simulink library "Word_Multiplexers_Lib"  (Simulink 8.7)
settings: Solver=ode45  StartTime=0.0  StopTime=10.0  RelTol=1e-3
(part 3 of 3)

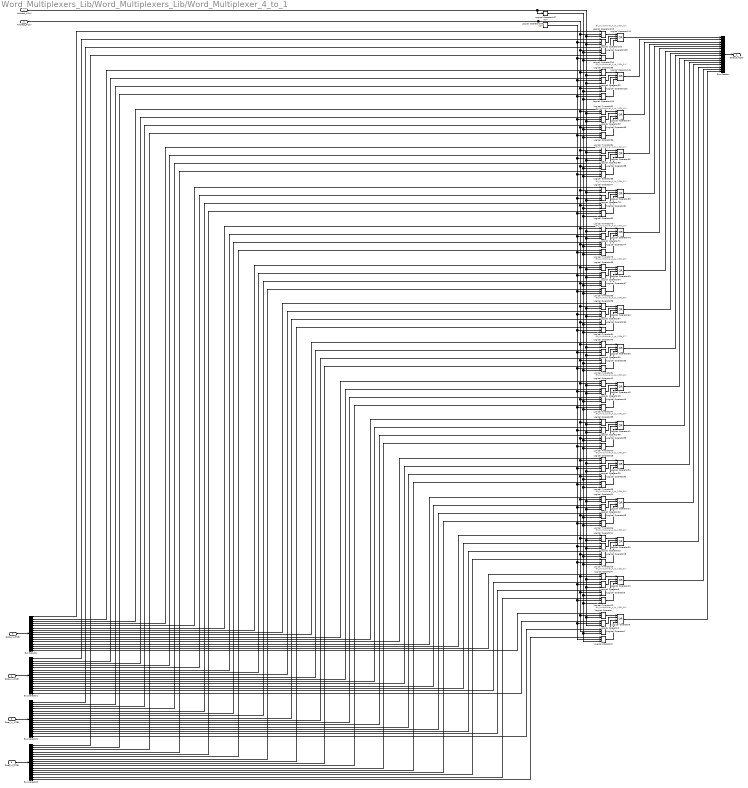
== system Word_Multiplexers_Lib/Word_Multiplexers_Lib/Word_Multiplexer_4_to_1 ==
  note: Bit_Multiplexer_4_to_1(Bit_15)
  note: Bit_Multiplexer_4_to_1(Bit_14)
  note: Bit_Multiplexer_4_to_1(Bit_13)
  note: Bit_Multiplexer_4_to_1(Bit_12)
  note: Bit_Multiplexer_4_to_1(Bit_11)
  note: Bit_Multiplexer_4_to_1(Bit_10)
  note: Bit_Multiplexer_4_to_1(Bit_09)
  note: Bit_Multiplexer_4_to_1(Bit_08)
  note: Bit_Multiplexer_4_to_1(Bit_07)
  note: Bit_Multiplexer_4_to_1(Bit_06)
  note: Bit_Multiplexer_4_to_1(Bit_05)
  note: Bit_Multiplexer_4_to_1(Bit_04)
  note: Bit_Multiplexer_4_to_1(Bit_03)
  note: Bit_Multiplexer_4_to_1(Bit_02)
  note: Bit_Multiplexer_4_to_1(Bit_01)
  note: Bit_Multiplexer_4_to_1(Bit_00)
  Address_1(1b) : Inport
  Address_0(1b) : Inport  Port=2
  Data_In_3(2B) : Inport  Port=3
  Data_In_2(2B) : Inport  Port=4
  Data_In_1(2B) : Inport  Port=5
  Data_In_0(2B) : Inport  Port=6
  Bus Creator : BusCreator  Inputs=16
  Bus Selector{,1..3} (4 alike) : BusSelector  OutputSignals=signal1,signal2,signal3,signal4,signal5,signal6,signal7,signal8,signal9,signal10,signal11,signal12,signal13,signal14,signal15,signal16
  Logical Operator{,1..5,9..10,14..15,18..19,21..22,25..26,28..29,32..33,35..36,39..40,42..43,46..47,49..50,53..54,56..57,60..61,63..64,67..68,70..71,74..75,77..78,81..82,84..85,88..89,91..92,95..96,98..99,102..103,105..106,109..110} (64 alike) : Logic  Inputs=3  IconShape=distinctive  AllPortsSameDT=off  OutDataTypeStr=boolean
  Logical Operator{8,13,20,27,34,41,48,55,62,69,76,83,90,97,104,111} (16 alike) : Logic  Operator=OR  Inputs=4  IconShape=distinctive  OutDataTypeStr=boolean
  Logical Operator107 : Logic  Operator=NOT  Inputs=4  IconShape=distinctive  AllPortsSameDT=off  OutDataTypeStr=boolean
  Logical Operator108 : Logic  Operator=NOT  Inputs=4  IconShape=distinctive  AllPortsSameDT=off  OutDataTypeStr=boolean
  Data_Out(2B) : Outport
  wires:
  Bus Creator/1 -> Data_Out(2B)/1
  Logical Operator34/1 -> Bus Creator/12
  Logical Operator41/1 -> Bus Creator/11
  Logical Operator48/1 -> Bus Creator/10
  Logical Operator55/1 -> Bus Creator/9
  Logical Operator27/1 -> Bus Creator/13
  Logical Operator20/1 -> Bus Creator/14
  Logical Operator13/1 -> Bus Creator/15
  Logical Operator8/1 -> Bus Creator/16
  Data_In_3(2B)/1 -> Bus Selector/1
  Data_In_2(2B)/1 -> Bus Selector1/1
  Data_In_1(2B)/1 -> Bus Selector2/1
  Data_In_0(2B)/1 -> Bus Selector3/1
  Logical Operator62/1 -> Bus Creator/8
  Logical Operator69/1 -> Bus Creator/7
  Logical Operator76/1 -> Bus Creator/6
  Logical Operator83/1 -> Bus Creator/5
  Logical Operator90/1 -> Bus Creator/4
  Logical Operator97/1 -> Bus Creator/3
  Logical Operator104/1 -> Bus Creator/2
  Logical Operator111/1 -> Bus Creator/1
  Logical Operator108/1 -> Logical Operator106/2, Logical Operator57/2, Logical Operator43/2, Logical Operator1/2, Logical Operator3/2, Logical Operator10/2, Logical Operator5/2, Logical Operator19/2, Logical Operator15/2, Logical Operator26/2, Logical Operator22/2, Logical Operator33/2, Logical Operator29/2, Logical Operator40/2, Logical Operator36/2, Logical Operator47/2, Logical Operator54/2, Logical Operator50/2, Logical Operator61/2, Logical Operator68/2, Logical Operator64/2, Logical Operator75/2, Logical Operator71/2, Logical Operator82/2, Logical Operator78/2, Logical Operator89/2, Logical Operator85/2, Logical Operator96/2, Logical Operator92/2, Logical Operator103/2, Logical Operator99/2, Logical Operator110/2
  Logical Operator107/1 -> Logical Operator109/3, Logical Operator60/3, Logical Operator46/3, Logical Operator10/3, Logical Operator2/3, Logical Operator3/3, Logical Operator9/3, Logical Operator19/3, Logical Operator18/3, Logical Operator26/3, Logical Operator25/3, Logical Operator33/3, Logical Operator32/3, Logical Operator40/3, Logical Operator39/3, Logical Operator47/3, Logical Operator54/3, Logical Operator53/3, Logical Operator61/3, Logical Operator68/3, Logical Operator67/3, Logical Operator75/3, Logical Operator74/3, Logical Operator82/3, Logical Operator81/3, Logical Operator89/3, Logical Operator88/3, Logical Operator96/3, Logical Operator95/3, Logical Operator103/3, Logical Operator102/3, Logical Operator110/3
  Bus Selector/16 -> Logical Operator/1  "<signal16>"
  Bus Selector1/16 -> Logical Operator1/1  "<signal16>"
  Bus Selector2/16 -> Logical Operator2/1  "<signal16>"
  Bus Selector3/16 -> Logical Operator3/1  "<signal16>"
  Logical Operator3/1 -> Logical Operator8/4
  Logical Operator2/1 -> Logical Operator8/3
  Logical Operator1/1 -> Logical Operator8/2
  Logical Operator/1 -> Logical Operator8/1
  Bus Selector/15 -> Logical Operator4/1  "<signal15>"
  Bus Selector1/15 -> Logical Operator5/1  "<signal15>"
  Bus Selector2/15 -> Logical Operator9/1  "<signal15>"
  Bus Selector3/15 -> Logical Operator10/1  "<signal15>"
  Logical Operator10/1 -> Logical Operator13/4
  Logical Operator9/1 -> Logical Operator13/3
  Logical Operator5/1 -> Logical Operator13/2
  Logical Operator4/1 -> Logical Operator13/1
  Bus Selector/14 -> Logical Operator14/1  "<signal14>"
  Bus Selector1/14 -> Logical Operator15/1  "<signal14>"
  Bus Selector2/14 -> Logical Operator18/1  "<signal14>"
  Bus Selector3/14 -> Logical Operator19/1  "<signal14>"
  Logical Operator19/1 -> Logical Operator20/4
  Logical Operator18/1 -> Logical Operator20/3
  Logical Operator15/1 -> Logical Operator20/2
  Logical Operator14/1 -> Logical Operator20/1
  Bus Selector/13 -> Logical Operator21/1  "<signal13>"
  Bus Selector1/13 -> Logical Operator22/1  "<signal13>"
  Bus Selector2/13 -> Logical Operator25/1  "<signal13>"
  Bus Selector3/13 -> Logical Operator26/1  "<signal13>"
  Logical Operator26/1 -> Logical Operator27/4
  Logical Operator25/1 -> Logical Operator27/3
  Logical Operator22/1 -> Logical Operator27/2
  Logical Operator21/1 -> Logical Operator27/1
  Bus Selector/12 -> Logical Operator28/1  "<signal12>"
  Bus Selector1/12 -> Logical Operator29/1  "<signal12>"
  Bus Selector2/12 -> Logical Operator32/1  "<signal12>"
  Bus Selector3/12 -> Logical Operator33/1  "<signal12>"
  Logical Operator33/1 -> Logical Operator34/4
  Logical Operator32/1 -> Logical Operator34/3
  Logical Operator29/1 -> Logical Operator34/2
  Logical Operator28/1 -> Logical Operator34/1
  Bus Selector/11 -> Logical Operator35/1  "<signal11>"
  Bus Selector1/11 -> Logical Operator36/1  "<signal11>"
  Bus Selector2/11 -> Logical Operator39/1  "<signal11>"
  Bus Selector3/11 -> Logical Operator40/1  "<signal11>"
  Logical Operator40/1 -> Logical Operator41/4
  Logical Operator39/1 -> Logical Operator41/3
  Logical Operator36/1 -> Logical Operator41/2
  Logical Operator35/1 -> Logical Operator41/1
  Bus Selector/10 -> Logical Operator42/1  "<signal10>"
  Bus Selector1/10 -> Logical Operator43/1  "<signal10>"
  Bus Selector2/10 -> Logical Operator46/1  "<signal10>"
  Bus Selector3/10 -> Logical Operator47/1  "<signal10>"
  Logical Operator47/1 -> Logical Operator48/4
  Logical Operator46/1 -> Logical Operator48/3
  Logical Operator43/1 -> Logical Operator48/2
  Logical Operator42/1 -> Logical Operator48/1
  Bus Selector/9 -> Logical Operator49/1  "<signal9>"
  Bus Selector1/9 -> Logical Operator50/1  "<signal9>"
  Bus Selector2/9 -> Logical Operator53/1  "<signal9>"
  Bus Selector3/9 -> Logical Operator54/1  "<signal9>"
  Logical Operator54/1 -> Logical Operator55/4
  Logical Operator53/1 -> Logical Operator55/3
  Logical Operator50/1 -> Logical Operator55/2
  Logical Operator49/1 -> Logical Operator55/1
  Bus Selector/8 -> Logical Operator56/1  "<signal8>"
  Bus Selector1/8 -> Logical Operator57/1  "<signal8>"
  Bus Selector2/8 -> Logical Operator60/1  "<signal8>"
  Bus Selector3/8 -> Logical Operator61/1  "<signal8>"
  Logical Operator61/1 -> Logical Operator62/4
  Logical Operator60/1 -> Logical Operator62/3
  Logical Operator57/1 -> Logical Operator62/2
  Logical Operator56/1 -> Logical Operator62/1
  Bus Selector/7 -> Logical Operator63/1  "<signal7>"
  Bus Selector1/7 -> Logical Operator64/1  "<signal7>"
  Bus Selector2/7 -> Logical Operator67/1  "<signal7>"
  Bus Selector3/7 -> Logical Operator68/1  "<signal7>"
  Logical Operator68/1 -> Logical Operator69/4
  Logical Operator67/1 -> Logical Operator69/3
  Logical Operator64/1 -> Logical Operator69/2
  Logical Operator63/1 -> Logical Operator69/1
  Bus Selector/6 -> Logical Operator70/1  "<signal6>"
  Bus Selector1/6 -> Logical Operator71/1  "<signal6>"
  Bus Selector2/6 -> Logical Operator74/1  "<signal6>"
  Bus Selector3/6 -> Logical Operator75/1  "<signal6>"
  Logical Operator75/1 -> Logical Operator76/4
  Logical Operator74/1 -> Logical Operator76/3
  Logical Operator71/1 -> Logical Operator76/2
  Logical Operator70/1 -> Logical Operator76/1
  Bus Selector/5 -> Logical Operator77/1  "<signal5>"
  Bus Selector1/5 -> Logical Operator78/1  "<signal5>"
  Bus Selector2/5 -> Logical Operator81/1  "<signal5>"
  Bus Selector3/5 -> Logical Operator82/1  "<signal5>"
  Logical Operator82/1 -> Logical Operator83/4
  Logical Operator81/1 -> Logical Operator83/3
  Logical Operator78/1 -> Logical Operator83/2
  Logical Operator77/1 -> Logical Operator83/1
  Bus Selector/4 -> Logical Operator84/1  "<signal4>"
  Bus Selector1/4 -> Logical Operator85/1  "<signal4>"
  Bus Selector2/4 -> Logical Operator88/1  "<signal4>"
  Bus Selector3/4 -> Logical Operator89/1  "<signal4>"
  Logical Operator89/1 -> Logical Operator90/4
  Logical Operator88/1 -> Logical Operator90/3
  Logical Operator85/1 -> Logical Operator90/2
  Logical Operator84/1 -> Logical Operator90/1
  Bus Selector/3 -> Logical Operator91/1  "<signal3>"
  Bus Selector1/3 -> Logical Operator92/1  "<signal3>"
  Bus Selector2/3 -> Logical Operator95/1  "<signal3>"
  Bus Selector3/3 -> Logical Operator96/1  "<signal3>"
  Logical Operator96/1 -> Logical Operator97/4
  Logical Operator95/1 -> Logical Operator97/3
  Logical Operator92/1 -> Logical Operator97/2
  Logical Operator91/1 -> Logical Operator97/1
  Bus Selector/2 -> Logical Operator98/1  "<signal2>"
  Bus Selector1/2 -> Logical Operator99/1  "<signal2>"
  Bus Selector2/2 -> Logical Operator102/1  "<signal2>"
  Bus Selector3/2 -> Logical Operator103/1  "<signal2>"
  Logical Operator103/1 -> Logical Operator104/4
  Logical Operator102/1 -> Logical Operator104/3
  Logical Operator99/1 -> Logical Operator104/2
  Logical Operator98/1 -> Logical Operator104/1
  Address_0(1b)/1 -> Logical Operator105/2, Logical Operator56/2, Logical Operator42/2, Logical Operator/2, Logical Operator2/2, Logical Operator9/2, Logical Operator4/2, Logical Operator18/2, Logical Operator14/2, Logical Operator25/2, Logical Operator21/2, Logical Operator32/2, Logical Operator28/2, Logical Operator39/2, Logical Operator35/2, Logical Operator46/2, Logical Operator53/2, Logical Operator49/2, Logical Operator60/2, Logical Operator67/2, Logical Operator63/2, Logical Operator74/2, Logical Operator70/2, Logical Operator81/2, Logical Operator77/2, Logical Operator88/2, Logical Operator84/2, Logical Operator95/2, Logical Operator91/2, Logical Operator102/2, Logical Operator98/2, Logical Operator109/2, Logical Operator108/1
  Address_1(1b)/1 -> Logical Operator107/1, Logical Operator105/3, Logical Operator56/3, Logical Operator42/3, Logical Operator/3, Logical Operator1/3, Logical Operator5/3, Logical Operator4/3, Logical Operator15/3, Logical Operator14/3, Logical Operator22/3, Logical Operator21/3, Logical Operator29/3, Logical Operator28/3, Logical Operator36/3, Logical Operator35/3, Logical Operator43/3, Logical Operator50/3, Logical Operator49/3, Logical Operator57/3, Logical Operator64/3, Logical Operator63/3, Logical Operator71/3, Logical Operator70/3, Logical Operator78/3, Logical Operator77/3, Logical Operator85/3, Logical Operator84/3, Logical Operator92/3, Logical Operator91/3, Logical Operator99/3, Logical Operator98/3, Logical Operator106/3
  Bus Selector/1 -> Logical Operator105/1  "<signal1>"
  Bus Selector1/1 -> Logical Operator106/1  "<signal1>"
  Bus Selector2/1 -> Logical Operator109/1  "<signal1>"
  Bus Selector3/1 -> Logical Operator110/1  "<signal1>"
  Logical Operator110/1 -> Logical Operator111/4
  Logical Operator109/1 -> Logical Operator111/3
  Logical Operator106/1 -> Logical Operator111/2
  Logical Operator105/1 -> Logical Operator111/1

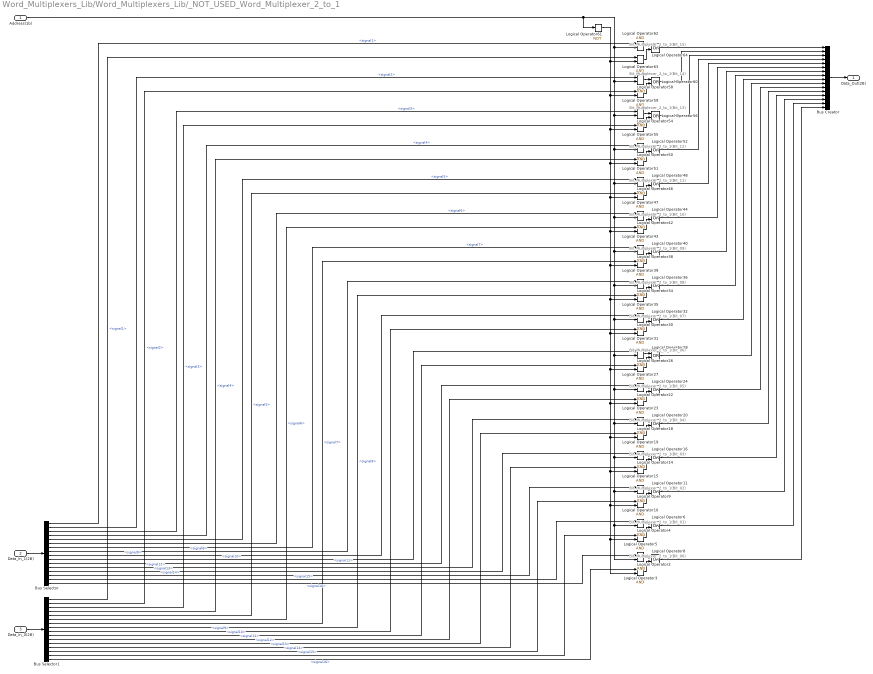
== system Word_Multiplexers_Lib/Word_Multiplexers_Lib/_NOT_USED_Word_Multiplexer_2_to_1 ==
  note: Bit_Multiplexer_2_to_1(Bit_15)
  note: Bit_Multiplexer_2_to_1(Bit_14)
  note: Bit_Multiplexer_2_to_1(Bit_13)
  note: Bit_Multiplexer_2_to_1(Bit_12)
  note: Bit_Multiplexer_2_to_1(Bit_11)
  note: Bit_Multiplexer_2_to_1(Bit_10)
  note: Bit_Multiplexer_2_to_1(Bit_09)
  note: Bit_Multiplexer_2_to_1(Bit_08)
  note: Bit_Multiplexer_2_to_1(Bit_07)
  note: Bit_Multiplexer_2_to_1(Bit_06)
  note: Bit_Multiplexer_2_to_1(Bit_05)
  note: Bit_Multiplexer_2_to_1(Bit_04)
  note: Bit_Multiplexer_2_to_1(Bit_03)
  note: Bit_Multiplexer_2_to_1(Bit_02)
  note: Bit_Multiplexer_2_to_1(Bit_01)
  note: Bit_Multiplexer_2_to_1(Bit_00)
  Address(1b) : Inport
  Data_In_1(2B) : Inport  Port=2
  Data_In_0(2B) : Inport  Port=3
  Bus Creator : BusCreator  Inputs=16
  Bus Selector : BusSelector  OutputSignals=signal1,signal2,signal3,signal4,signal5,signal6,signal7,signal8,signal9,signal10,signal11,signal12,signal13,signal14,signal15,signal16
  Bus Selector1 : BusSelector  OutputSignals=signal1,signal2,signal3,signal4,signal5,signal6,signal7,signal8,signal9,signal10,signal11,signal12,signal13,signal14,signal15,signal16
  Logical Operator{2..5,9..10,14..15,18..19,22..23,26..27,30..31,34..35,38..39,42..43,46..47,50..51,54..55,58..59,62..63} (32 alike) : Logic  IconShape=distinctive  AllPortsSameDT=off  OutDataTypeStr=boolean
  Logical Operator{6,8,11,16,20,24,28,32,36,40,44,48,52,56,60,64} (16 alike) : Logic  Operator=OR  IconShape=distinctive  OutDataTypeStr=boolean
  Logical Operator61 : Logic  Operator=NOT  Inputs=4  IconShape=distinctive  AllPortsSameDT=off  OutDataTypeStr=boolean
  Data_Out(2B) : Outport
  wires:
  Logical Operator64/1 -> Bus Creator/1
  Logical Operator60/1 -> Bus Creator/2
  Logical Operator56/1 -> Bus Creator/3
  Logical Operator52/1 -> Bus Creator/4
  Logical Operator48/1 -> Bus Creator/5
  Logical Operator44/1 -> Bus Creator/6
  Logical Operator40/1 -> Bus Creator/7
  Logical Operator36/1 -> Bus Creator/8
  Data_In_0(2B)/1 -> Bus Selector1/1
  Data_In_1(2B)/1 -> Bus Selector/1
  Logical Operator8/1 -> Bus Creator/16
  Logical Operator6/1 -> Bus Creator/15
  Logical Operator11/1 -> Bus Creator/14
  Logical Operator16/1 -> Bus Creator/13
  Logical Operator32/1 -> Bus Creator/9
  Logical Operator28/1 -> Bus Creator/10
  Logical Operator24/1 -> Bus Creator/11
  Logical Operator20/1 -> Bus Creator/12
  Bus Creator/1 -> Data_Out(2B)/1
  Logical Operator61/1 -> Logical Operator3/2, Logical Operator5/2, Logical Operator10/2, Logical Operator15/2, Logical Operator19/2, Logical Operator23/2, Logical Operator27/2, Logical Operator31/2, Logical Operator35/2, Logical Operator39/2, Logical Operator43/2, Logical Operator47/2, Logical Operator51/2, Logical Operator55/2, Logical Operator59/2, Logical Operator63/2
  Bus Selector/16 -> Logical Operator2/1  "<signal16>"
  Bus Selector1/16 -> Logical Operator3/1  "<signal16>"
  Logical Operator3/1 -> Logical Operator8/2
  Logical Operator2/1 -> Logical Operator8/1
  Bus Selector/15 -> Logical Operator4/1  "<signal15>"
  Bus Selector1/15 -> Logical Operator5/1  "<signal15>"
  Logical Operator5/1 -> Logical Operator6/2
  Logical Operator4/1 -> Logical Operator6/1
  Bus Selector/14 -> Logical Operator9/1  "<signal14>"
  Bus Selector1/14 -> Logical Operator10/1  "<signal14>"
  Logical Operator10/1 -> Logical Operator11/2
  Logical Operator9/1 -> Logical Operator11/1
  Bus Selector/13 -> Logical Operator14/1  "<signal13>"
  Bus Selector1/13 -> Logical Operator15/1  "<signal13>"
  Logical Operator15/1 -> Logical Operator16/2
  Logical Operator14/1 -> Logical Operator16/1
  Bus Selector/12 -> Logical Operator18/1  "<signal12>"
  Bus Selector1/12 -> Logical Operator19/1  "<signal12>"
  Logical Operator19/1 -> Logical Operator20/2
  Logical Operator18/1 -> Logical Operator20/1
  Bus Selector/11 -> Logical Operator22/1  "<signal11>"
  Bus Selector1/11 -> Logical Operator23/1  "<signal11>"
  Logical Operator23/1 -> Logical Operator24/2
  Logical Operator22/1 -> Logical Operator24/1
  Bus Selector/10 -> Logical Operator26/1  "<signal10>"
  Bus Selector1/10 -> Logical Operator27/1  "<signal10>"
  Logical Operator27/1 -> Logical Operator28/2
  Logical Operator26/1 -> Logical Operator28/1
  Bus Selector/9 -> Logical Operator30/1  "<signal9>"
  Bus Selector1/9 -> Logical Operator31/1  "<signal9>"
  Logical Operator31/1 -> Logical Operator32/2
  Logical Operator30/1 -> Logical Operator32/1
  Bus Selector/8 -> Logical Operator34/1  "<signal8>"
  Bus Selector1/8 -> Logical Operator35/1  "<signal8>"
  Logical Operator35/1 -> Logical Operator36/2
  Logical Operator34/1 -> Logical Operator36/1
  Bus Selector/7 -> Logical Operator38/1  "<signal7>"
  Bus Selector1/7 -> Logical Operator39/1  "<signal7>"
  Logical Operator39/1 -> Logical Operator40/2
  Logical Operator38/1 -> Logical Operator40/1
  Bus Selector/6 -> Logical Operator42/1  "<signal6>"
  Bus Selector1/6 -> Logical Operator43/1  "<signal6>"
  Logical Operator43/1 -> Logical Operator44/2
  Logical Operator42/1 -> Logical Operator44/1
  Bus Selector/5 -> Logical Operator46/1  "<signal5>"
  Bus Selector1/5 -> Logical Operator47/1  "<signal5>"
  Logical Operator47/1 -> Logical Operator48/2
  Logical Operator46/1 -> Logical Operator48/1
  Bus Selector/4 -> Logical Operator50/1  "<signal4>"
  Bus Selector1/4 -> Logical Operator51/1  "<signal4>"
  Logical Operator51/1 -> Logical Operator52/2
  Logical Operator50/1 -> Logical Operator52/1
  Bus Selector/3 -> Logical Operator54/1  "<signal3>"
  Bus Selector1/3 -> Logical Operator55/1  "<signal3>"
  Logical Operator55/1 -> Logical Operator56/2
  Logical Operator54/1 -> Logical Operator56/1
  Bus Selector/2 -> Logical Operator58/1  "<signal2>"
  Bus Selector1/2 -> Logical Operator59/1  "<signal2>"
  Logical Operator59/1 -> Logical Operator60/2
  Logical Operator58/1 -> Logical Operator60/1
  Address(1b)/1 -> Logical Operator22/2, Logical Operator18/2, Logical Operator2/2, Logical Operator4/2, Logical Operator9/2, Logical Operator14/2, Logical Operator26/2, Logical Operator30/2, Logical Operator34/2, Logical Operator38/2, Logical Operator42/2, Logical Operator46/2, Logical Operator50/2, Logical Operator54/2, Logical Operator58/2, Logical Operator62/2, Logical Operator61/1
  Bus Selector/1 -> Logical Operator62/1  "<signal1>"
  Bus Selector1/1 -> Logical Operator63/1  "<signal1>"
  Logical Operator63/1 -> Logical Operator64/2
  Logical Operator62/1 -> Logical Operator64/1

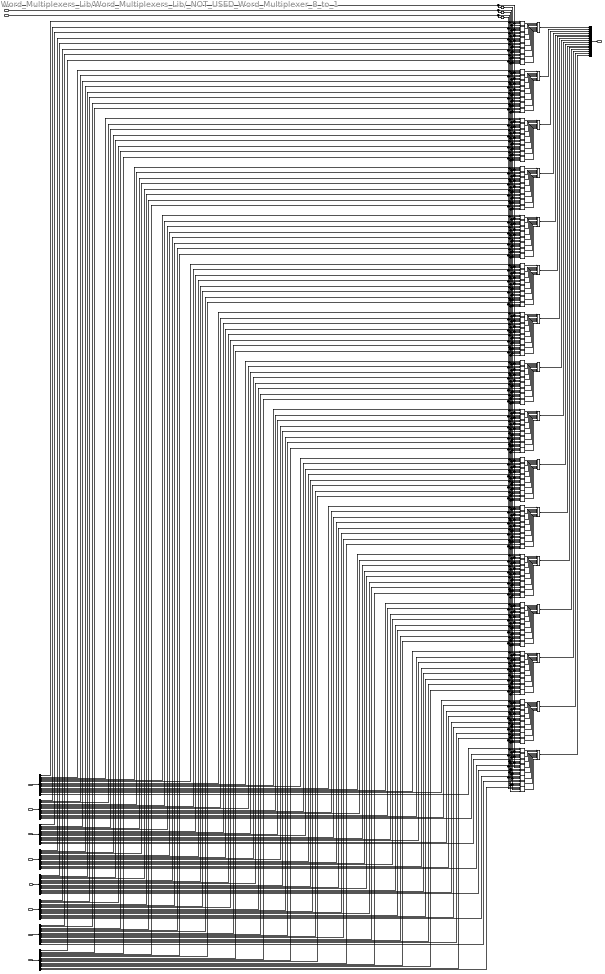
== system Word_Multiplexers_Lib/Word_Multiplexers_Lib/_NOT_USED_Word_Multiplexer_8_to_1 ==
  note: Bit_Multiplexer_8_to_1(Bit_15)
  note: Bit_Multiplexer_8_to_1(Bit_14)
  note: Bit_Multiplexer_8_to_1(Bit_13)
  note: Bit_Multiplexer_8_to_1(Bit_12)
  note: Bit_Multiplexer_8_to_1(Bit_11)
  note: Bit_Multiplexer_8_to_1(Bit_10)
  note: Bit_Multiplexer_8_to_1(Bit_09)
  note: Bit_Multiplexer_8_to_1(Bit_08)
  note: Bit_Multiplexer_8_to_1(Bit_07)
  note: Bit_Multiplexer_8_to_1(Bit_06)
  note: Bit_Multiplexer_8_to_1(Bit_05)
  note: Bit_Multiplexer_8_to_1(Bit_04)
  note: Bit_Multiplexer_8_to_1(Bit_03)
  note: Bit_Multiplexer_8_to_1(Bit_02)
  note: Bit_Multiplexer_8_to_1(Bit_01)
  note: Bit_Multiplexer_8_to_1(Bit_00)
  Address_2(1b) : Inport
  Address_1(1b) : Inport  Port=2
  Address_0(1b) : Inport  Port=3
  Data_In_7(2B) : Inport  Port=4
  Data_In_6(2B) : Inport  Port=5
  Data_In_5(2B) : Inport  Port=6
  Data_In_4(2B) : Inport  Port=7
  Data_In_3(2B) : Inport  Port=8
  Data_In_2(2B) : Inport  Port=9
  Data_In_1(2B) : Inport  Port=10
  Data_In_0(2B) : Inport  Port=11
  Bus Creator : BusCreator  Inputs=16
  Bus Selector{,1..7} (8 alike) : BusSelector  OutputSignals=signal1,signal2,signal3,signal4,signal5,signal6,signal7,signal8,signal9,signal10,signal11,signal12,signal13,signal14,signal15,signal16
  Logical Operator{,1..7,9,13,17..22,24..25,29..34,36..37,41..46,48..49,53..58,60..61,65..70,72..73,77..82,84..85,89..94,96..97,101..106,108..109,113..118,120..121,125..130,132..133,137..142,144..145,149..154,156..157,161..166,168..169,173..178,180..181,185..190} (128 alike) : Logic  Inputs=4  IconShape=distinctive  AllPortsSameDT=off  OutDataTypeStr=boolean
  Logical Operator{8,23,35,47,59,71,83,95,107,119,131,143,155,167,179,191} (16 alike) : Logic  Operator=OR  Inputs=8  IconShape=distinctive  OutDataTypeStr=boolean
  Logical Operator182 : Logic  Operator=NOT  Inputs=4  IconShape=distinctive  AllPortsSameDT=off  OutDataTypeStr=boolean
  Logical Operator183 : Logic  Operator=NOT  Inputs=4  IconShape=distinctive  AllPortsSameDT=off  OutDataTypeStr=boolean
  Logical Operator184 : Logic  Operator=NOT  Inputs=4  IconShape=distinctive  AllPortsSameDT=off  OutDataTypeStr=boolean
  Data_Out(2B) : Outport
  wires:
  Logical Operator59/1 -> Bus Creator/12
  Logical Operator71/1 -> Bus Creator/11
  Logical Operator83/1 -> Bus Creator/10
  Logical Operator95/1 -> Bus Creator/9
  Logical Operator47/1 -> Bus Creator/13
  Logical Operator35/1 -> Bus Creator/14
  Logical Operator23/1 -> Bus Creator/15
  Logical Operator8/1 -> Bus Creator/16
  Bus Creator/1 -> Data_Out(2B)/1
  Data_In_7(2B)/1 -> Bus Selector/1
  Data_In_6(2B)/1 -> Bus Selector1/1
  Data_In_5(2B)/1 -> Bus Selector2/1
  Data_In_4(2B)/1 -> Bus Selector3/1
  Data_In_3(2B)/1 -> Bus Selector4/1
  Data_In_2(2B)/1 -> Bus Selector5/1
  Data_In_1(2B)/1 -> Bus Selector6/1
  Data_In_0(2B)/1 -> Bus Selector7/1
  Logical Operator155/1 -> Bus Creator/4
  Logical Operator167/1 -> Bus Creator/3
  Logical Operator179/1 -> Bus Creator/2
  Logical Operator191/1 -> Bus Creator/1
  Logical Operator143/1 -> Bus Creator/5
  Logical Operator131/1 -> Bus Creator/6
  Logical Operator119/1 -> Bus Creator/7
  Logical Operator107/1 -> Bus Creator/8
  Logical Operator184/1 -> Logical Operator181/2, Logical Operator186/2, Logical Operator188/2, Logical Operator190/2, Logical Operator121/2, Logical Operator126/2, Logical Operator128/2, Logical Operator85/2, Logical Operator90/2, Logical Operator92/2, Logical Operator1/2, Logical Operator3/2, Logical Operator5/2, Logical Operator7/2, Logical Operator22/2, Logical Operator20/2, Logical Operator18/2, Logical Operator13/2, Logical Operator34/2, Logical Operator32/2, Logical Operator30/2, Logical Operator25/2, Logical Operator46/2, Logical Operator44/2, Logical Operator42/2, Logical Operator37/2, Logical Operator58/2, Logical Operator56/2, Logical Operator54/2, Logical Operator49/2, Logical Operator70/2, Logical Operator68/2, Logical Operator66/2, Logical Operator61/2, Logical Operator82/2, Logical Operator80/2, Logical Operator78/2, Logical Operator73/2, Logical Operator94/2, Logical Operator106/2, Logical Operator104/2, Logical Operator102/2, Logical Operator97/2, Logical Operator118/2, Logical Operator116/2, Logical Operator114/2, Logical Operator109/2, Logical Operator130/2, Logical Operator142/2, Logical Operator140/2, Logical Operator138/2, Logical Operator133/2, Logical Operator154/2, Logical Operator152/2, Logical Operator150/2, Logical Operator145/2, Logical Operator166/2, Logical Operator164/2, Logical Operator162/2, Logical Operator157/2, Logical Operator178/2, Logical Operator176/2, Logical Operator174/2, Logical Operator169/2
  Logical Operator183/1 -> Logical Operator185/4, Logical Operator186/4, Logical Operator189/4, Logical Operator190/4, Logical Operator125/4, Logical Operator126/4, Logical Operator129/4, Logical Operator89/4, Logical Operator90/4, Logical Operator93/4, Logical Operator2/4, Logical Operator3/4, Logical Operator6/4, Logical Operator7/4, Logical Operator22/4, Logical Operator21/4, Logical Operator18/4, Logical Operator17/4, Logical Operator34/4, Logical Operator33/4, Logical Operator30/4, Logical Operator29/4, Logical Operator46/4, Logical Operator45/4, Logical Operator42/4, Logical Operator41/4, Logical Operator58/4, Logical Operator57/4, Logical Operator54/4, Logical Operator53/4, Logical Operator70/4, Logical Operator69/4, Logical Operator66/4, Logical Operator65/4, Logical Operator82/4, Logical Operator81/4, Logical Operator78/4, Logical Operator77/4, Logical Operator94/4, Logical Operator106/4, Logical Operator105/4, Logical Operator102/4, Logical Operator101/4, Logical Operator118/4, Logical Operator117/4, Logical Operator114/4, Logical Operator113/4, Logical Operator130/4, Logical Operator142/4, Logical Operator141/4, Logical Operator138/4, Logical Operator137/4, Logical Operator154/4, Logical Operator153/4, Logical Operator150/4, Logical Operator149/4, Logical Operator166/4, Logical Operator165/4, Logical Operator162/4, Logical Operator161/4, Logical Operator178/4, Logical Operator177/4, Logical Operator174/4, Logical Operator173/4
  Logical Operator182/1 -> Logical Operator187/3, Logical Operator188/3, Logical Operator189/3, Logical Operator190/3, Logical Operator127/3, Logical Operator128/3, Logical Operator129/3, Logical Operator91/3, Logical Operator92/3, Logical Operator93/3, Logical Operator4/3, Logical Operator5/3, Logical Operator6/3, Logical Operator7/3, Logical Operator22/3, Logical Operator21/3, Logical Operator20/3, Logical Operator19/3, Logical Operator34/3, Logical Operator33/3, Logical Operator32/3, Logical Operator31/3, Logical Operator46/3, Logical Operator45/3, Logical Operator44/3, Logical Operator43/3, Logical Operator58/3, Logical Operator57/3, Logical Operator56/3, Logical Operator55/3, Logical Operator70/3, Logical Operator69/3, Logical Operator68/3, Logical Operator67/3, Logical Operator82/3, Logical Operator81/3, Logical Operator80/3, Logical Operator79/3, Logical Operator94/3, Logical Operator106/3, Logical Operator105/3, Logical Operator104/3, Logical Operator103/3, Logical Operator118/3, Logical Operator117/3, Logical Operator116/3, Logical Operator115/3, Logical Operator130/3, Logical Operator142/3, Logical Operator141/3, Logical Operator140/3, Logical Operator139/3, Logical Operator154/3, Logical Operator153/3, Logical Operator152/3, Logical Operator151/3, Logical Operator166/3, Logical Operator165/3, Logical Operator164/3, Logical Operator163/3, Logical Operator178/3, Logical Operator177/3, Logical Operator176/3, Logical Operator175/3
  Bus Selector/16 -> Logical Operator/1  "<signal16>"
  Bus Selector1/16 -> Logical Operator1/1  "<signal16>"
  Bus Selector2/16 -> Logical Operator2/1  "<signal16>"
  Bus Selector3/16 -> Logical Operator3/1  "<signal16>"
  Bus Selector4/16 -> Logical Operator4/1  "<signal16>"
  Bus Selector5/16 -> Logical Operator5/1  "<signal16>"
  Bus Selector6/16 -> Logical Operator6/1  "<signal16>"
  Bus Selector7/16 -> Logical Operator7/1  "<signal16>"
  Logical Operator7/1 -> Logical Operator8/8
  Logical Operator6/1 -> Logical Operator8/7
  Logical Operator5/1 -> Logical Operator8/6
  Logical Operator4/1 -> Logical Operator8/5
  Logical Operator3/1 -> Logical Operator8/4
  Logical Operator2/1 -> Logical Operator8/3
  Logical Operator1/1 -> Logical Operator8/2
  Logical Operator/1 -> Logical Operator8/1
  Bus Selector/15 -> Logical Operator9/1  "<signal15>"
  Bus Selector1/15 -> Logical Operator13/1  "<signal15>"
  Bus Selector2/15 -> Logical Operator17/1  "<signal15>"
  Bus Selector3/15 -> Logical Operator18/1  "<signal15>"
  Bus Selector4/15 -> Logical Operator19/1  "<signal15>"
  Bus Selector5/15 -> Logical Operator20/1  "<signal15>"
  Bus Selector6/15 -> Logical Operator21/1  "<signal15>"
  Bus Selector7/15 -> Logical Operator22/1  "<signal15>"
  Logical Operator22/1 -> Logical Operator23/8
  Logical Operator21/1 -> Logical Operator23/7
  Logical Operator20/1 -> Logical Operator23/6
  Logical Operator19/1 -> Logical Operator23/5
  Logical Operator18/1 -> Logical Operator23/4
  Logical Operator17/1 -> Logical Operator23/3
  Logical Operator13/1 -> Logical Operator23/2
  Logical Operator9/1 -> Logical Operator23/1
  Bus Selector/14 -> Logical Operator24/1  "<signal14>"
  Bus Selector1/14 -> Logical Operator25/1  "<signal14>"
  Bus Selector2/14 -> Logical Operator29/1  "<signal14>"
  Bus Selector3/14 -> Logical Operator30/1  "<signal14>"
  Bus Selector4/14 -> Logical Operator31/1  "<signal14>"
  Bus Selector5/14 -> Logical Operator32/1  "<signal14>"
  Bus Selector6/14 -> Logical Operator33/1  "<signal14>"
  Bus Selector7/14 -> Logical Operator34/1  "<signal14>"
  Logical Operator34/1 -> Logical Operator35/8
  Logical Operator33/1 -> Logical Operator35/7
  Logical Operator32/1 -> Logical Operator35/6
  Logical Operator31/1 -> Logical Operator35/5
  Logical Operator30/1 -> Logical Operator35/4
  Logical Operator29/1 -> Logical Operator35/3
  Logical Operator25/1 -> Logical Operator35/2
  Logical Operator24/1 -> Logical Operator35/1
  Bus Selector/13 -> Logical Operator36/1  "<signal13>"
  Bus Selector1/13 -> Logical Operator37/1  "<signal13>"
  Bus Selector2/13 -> Logical Operator41/1  "<signal13>"
  Bus Selector3/13 -> Logical Operator42/1  "<signal13>"
  Bus Selector4/13 -> Logical Operator43/1  "<signal13>"
  Bus Selector5/13 -> Logical Operator44/1  "<signal13>"
  Bus Selector6/13 -> Logical Operator45/1  "<signal13>"
  Bus Selector7/13 -> Logical Operator46/1  "<signal13>"
  Logical Operator46/1 -> Logical Operator47/8
  Logical Operator45/1 -> Logical Operator47/7
  Logical Operator44/1 -> Logical Operator47/6
  Logical Operator43/1 -> Logical Operator47/5
  Logical Operator42/1 -> Logical Operator47/4
  Logical Operator41/1 -> Logical Operator47/3
  Logical Operator37/1 -> Logical Operator47/2
  Logical Operator36/1 -> Logical Operator47/1
  Bus Selector/12 -> Logical Operator48/1  "<signal12>"
  Bus Selector1/12 -> Logical Operator49/1  "<signal12>"
  Bus Selector2/12 -> Logical Operator53/1  "<signal12>"
  Bus Selector3/12 -> Logical Operator54/1  "<signal12>"
  Bus Selector4/12 -> Logical Operator55/1  "<signal12>"
  Bus Selector5/12 -> Logical Operator56/1  "<signal12>"
  Bus Selector6/12 -> Logical Operator57/1  "<signal12>"
  Bus Selector7/12 -> Logical Operator58/1  "<signal12>"
  Logical Operator58/1 -> Logical Operator59/8
  Logical Operator57/1 -> Logical Operator59/7
  Logical Operator56/1 -> Logical Operator59/6
  Logical Operator55/1 -> Logical Operator59/5
  Logical Operator54/1 -> Logical Operator59/4
  Logical Operator53/1 -> Logical Operator59/3
  Logical Operator49/1 -> Logical Operator59/2
  Logical Operator48/1 -> Logical Operator59/1
  Bus Selector/11 -> Logical Operator60/1  "<signal11>"
  Bus Selector1/11 -> Logical Operator61/1  "<signal11>"
  Bus Selector2/11 -> Logical Operator65/1  "<signal11>"
  Bus Selector3/11 -> Logical Operator66/1  "<signal11>"
  Bus Selector4/11 -> Logical Operator67/1  "<signal11>"
  Bus Selector5/11 -> Logical Operator68/1  "<signal11>"
  Bus Selector6/11 -> Logical Operator69/1  "<signal11>"
  Bus Selector7/11 -> Logical Operator70/1  "<signal11>"
  Logical Operator70/1 -> Logical Operator71/8
  Logical Operator69/1 -> Logical Operator71/7
  Logical Operator68/1 -> Logical Operator71/6
  Logical Operator67/1 -> Logical Operator71/5
  Logical Operator66/1 -> Logical Operator71/4
  Logical Operator65/1 -> Logical Operator71/3
  Logical Operator61/1 -> Logical Operator71/2
  Logical Operator60/1 -> Logical Operator71/1
  Bus Selector/10 -> Logical Operator72/1  "<signal10>"
  Bus Selector1/10 -> Logical Operator73/1  "<signal10>"
  Bus Selector2/10 -> Logical Operator77/1  "<signal10>"
  Bus Selector3/10 -> Logical Operator78/1  "<signal10>"
  Bus Selector4/10 -> Logical Operator79/1  "<signal10>"
  Bus Selector5/10 -> Logical Operator80/1  "<signal10>"
  Bus Selector6/10 -> Logical Operator81/1  "<signal10>"
  Bus Selector7/10 -> Logical Operator82/1  "<signal10>"
  Logical Operator82/1 -> Logical Operator83/8
  Logical Operator81/1 -> Logical Operator83/7
  Logical Operator80/1 -> Logical Operator83/6
  Logical Operator79/1 -> Logical Operator83/5
  Logical Operator78/1 -> Logical Operator83/4
  Logical Operator77/1 -> Logical Operator83/3
  Logical Operator73/1 -> Logical Operator83/2
  Logical Operator72/1 -> Logical Operator83/1
  Bus Selector/9 -> Logical Operator84/1  "<signal9>"
  Bus Selector1/9 -> Logical Operator85/1  "<signal9>"
  Bus Selector2/9 -> Logical Operator89/1  "<signal9>"
  Bus Selector3/9 -> Logical Operator90/1  "<signal9>"
  Bus Selector4/9 -> Logical Operator91/1  "<signal9>"
  Bus Selector5/9 -> Logical Operator92/1  "<signal9>"
  Bus Selector6/9 -> Logical Operator93/1  "<signal9>"
  Bus Selector7/9 -> Logical Operator94/1  "<signal9>"
  Logical Operator94/1 -> Logical Operator95/8
  Logical Operator93/1 -> Logical Operator95/7
  Logical Operator92/1 -> Logical Operator95/6
  Logical Operator91/1 -> Logical Operator95/5
  Logical Operator90/1 -> Logical Operator95/4
  Logical Operator89/1 -> Logical Operator95/3
  Logical Operator85/1 -> Logical Operator95/2
  Logical Operator84/1 -> Logical Operator95/1
  Bus Selector/8 -> Logical Operator96/1  "<signal8>"
  Bus Selector1/8 -> Logical Operator97/1  "<signal8>"
  Bus Selector2/8 -> Logical Operator101/1  "<signal8>"
  Bus Selector3/8 -> Logical Operator102/1  "<signal8>"
  Bus Selector4/8 -> Logical Operator103/1  "<signal8>"
  Bus Selector5/8 -> Logical Operator104/1  "<signal8>"
  Bus Selector6/8 -> Logical Operator105/1  "<signal8>"
  Bus Selector7/8 -> Logical Operator106/1  "<signal8>"
  Logical Operator106/1 -> Logical Operator107/8
  Logical Operator105/1 -> Logical Operator107/7
  Logical Operator104/1 -> Logical Operator107/6
  Logical Operator103/1 -> Logical Operator107/5
  Logical Operator102/1 -> Logical Operator107/4
  Logical Operator101/1 -> Logical Operator107/3
  Logical Operator97/1 -> Logical Operator107/2
  Logical Operator96/1 -> Logical Operator107/1
  Bus Selector/7 -> Logical Operator108/1  "<signal7>"
  Bus Selector1/7 -> Logical Operator109/1  "<signal7>"
  Bus Selector2/7 -> Logical Operator113/1  "<signal7>"
  Bus Selector3/7 -> Logical Operator114/1  "<signal7>"
  Bus Selector4/7 -> Logical Operator115/1  "<signal7>"
  Bus Selector5/7 -> Logical Operator116/1  "<signal7>"
  Bus Selector6/7 -> Logical Operator117/1  "<signal7>"
  Bus Selector7/7 -> Logical Operator118/1  "<signal7>"
  Logical Operator118/1 -> Logical Operator119/8
  Logical Operator117/1 -> Logical Operator119/7
  Logical Operator116/1 -> Logical Operator119/6
  Logical Operator115/1 -> Logical Operator119/5
  Logical Operator114/1 -> Logical Operator119/4
  Logical Operator113/1 -> Logical Operator119/3
  Logical Operator109/1 -> Logical Operator119/2
  Logical Operator108/1 -> Logical Operator119/1
  Bus Selector/6 -> Logical Operator120/1  "<signal6>"
  Bus Selector1/6 -> Logical Operator121/1  "<signal6>"
  Bus Selector2/6 -> Logical Operator125/1  "<signal6>"
  Bus Selector3/6 -> Logical Operator126/1  "<signal6>"
  Bus Selector4/6 -> Logical Operator127/1  "<signal6>"
  Bus Selector5/6 -> Logical Operator128/1  "<signal6>"
  Bus Selector6/6 -> Logical Operator129/1  "<signal6>"
  Bus Selector7/6 -> Logical Operator130/1  "<signal6>"
  Logical Operator130/1 -> Logical Operator131/8
  Logical Operator129/1 -> Logical Operator131/7
  Logical Operator128/1 -> Logical Operator131/6
  Logical Operator127/1 -> Logical Operator131/5
  Logical Operator126/1 -> Logical Operator131/4
  Logical Operator125/1 -> Logical Operator131/3
  Logical Operator121/1 -> Logical Operator131/2
  Logical Operator120/1 -> Logical Operator131/1
  Bus Selector/5 -> Logical Operator132/1  "<signal5>"
  Bus Selector1/5 -> Logical Operator133/1  "<signal5>"
  Bus Selector2/5 -> Logical Operator137/1  "<signal5>"
  Bus Selector3/5 -> Logical Operator138/1  "<signal5>"
  Bus Selector4/5 -> Logical Operator139/1  "<signal5>"
  Bus Selector5/5 -> Logical Operator140/1  "<signal5>"
  Bus Selector6/5 -> Logical Operator141/1  "<signal5>"
  Bus Selector7/5 -> Logical Operator142/1  "<signal5>"
  Logical Operator142/1 -> Logical Operator143/8
  Logical Operator141/1 -> Logical Operator143/7
  Logical Operator140/1 -> Logical Operator143/6
  Logical Operator139/1 -> Logical Operator143/5
  Logical Operator138/1 -> Logical Operator143/4
  Logical Operator137/1 -> Logical Operator143/3
  Logical Operator133/1 -> Logical Operator143/2
  Logical Operator132/1 -> Logical Operator143/1
  Bus Selector/4 -> Logical Operator144/1  "<signal4>"
  Bus Selector1/4 -> Logical Operator145/1  "<signal4>"
  Bus Selector2/4 -> Logical Operator149/1  "<signal4>"
  Bus Selector3/4 -> Logical Operator150/1  "<signal4>"
  Bus Selector4/4 -> Logical Operator151/1  "<signal4>"
  Bus Selector5/4 -> Logical Operator152/1  "<signal4>"
  Bus Selector6/4 -> Logical Operator153/1  "<signal4>"
  Bus Selector7/4 -> Logical Operator154/1  "<signal4>"
  Logical Operator154/1 -> Logical Operator155/8
  Logical Operator153/1 -> Logical Operator155/7
  Logical Operator152/1 -> Logical Operator155/6
  Logical Operator151/1 -> Logical Operator155/5
  Logical Operator150/1 -> Logical Operator155/4
  Logical Operator149/1 -> Logical Operator155/3
  Logical Operator145/1 -> Logical Operator155/2
  Logical Operator144/1 -> Logical Operator155/1
  Bus Selector/3 -> Logical Operator156/1  "<signal3>"
  Bus Selector1/3 -> Logical Operator157/1  "<signal3>"
  Bus Selector2/3 -> Logical Operator161/1  "<signal3>"
  Bus Selector3/3 -> Logical Operator162/1  "<signal3>"
  Bus Selector4/3 -> Logical Operator163/1  "<signal3>"
  Bus Selector5/3 -> Logical Operator164/1  "<signal3>"
  Bus Selector6/3 -> Logical Operator165/1  "<signal3>"
  Bus Selector7/3 -> Logical Operator166/1  "<signal3>"
  Logical Operator166/1 -> Logical Operator167/8
  Logical Operator165/1 -> Logical Operator167/7
  Logical Operator164/1 -> Logical Operator167/6
  Logical Operator163/1 -> Logical Operator167/5
  Logical Operator162/1 -> Logical Operator167/4
  Logical Operator161/1 -> Logical Operator167/3
  Logical Operator157/1 -> Logical Operator167/2
  Logical Operator156/1 -> Logical Operator167/1
  Bus Selector/2 -> Logical Operator168/1  "<signal2>"
  Bus Selector1/2 -> Logical Operator169/1  "<signal2>"
  Bus Selector2/2 -> Logical Operator173/1  "<signal2>"
  Bus Selector3/2 -> Logical Operator174/1  "<signal2>"
  Bus Selector4/2 -> Logical Operator175/1  "<signal2>"
  Bus Selector5/2 -> Logical Operator176/1  "<signal2>"
  Bus Selector6/2 -> Logical Operator177/1  "<signal2>"
  Bus Selector7/2 -> Logical Operator178/1  "<signal2>"
  Logical Operator178/1 -> Logical Operator179/8
  Logical Operator177/1 -> Logical Operator179/7
  Logical Operator176/1 -> Logical Operator179/6
  Logical Operator175/1 -> Logical Operator179/5
  Logical Operator174/1 -> Logical Operator179/4
  Logical Operator173/1 -> Logical Operator179/3
  Logical Operator169/1 -> Logical Operator179/2
  Logical Operator168/1 -> Logical Operator179/1
  Address_1(1b)/1 -> Logical Operator180/4, Logical Operator181/4, Logical Operator187/4, Logical Operator120/4, Logical Operator121/4, Logical Operator127/4, Logical Operator128/4, Logical Operator84/4, Logical Operator85/4, Logical Operator91/4, Logical Operator92/4, Logical Operator/4, Logical Operator1/4, Logical Operator4/4, Logical Operator5/4, Logical Operator20/4, Logical Operator19/4, Logical Operator13/4, Logical Operator9/4, Logical Operator32/4, Logical Operator31/4, Logical Operator25/4, Logical Operator24/4, Logical Operator44/4, Logical Operator43/4, Logical Operator37/4, Logical Operator36/4, Logical Operator56/4, Logical Operator55/4, Logical Operator49/4, Logical Operator48/4, Logical Operator68/4, Logical Operator67/4, Logical Operator61/4, Logical Operator60/4, Logical Operator80/4, Logical Operator79/4, Logical Operator73/4, Logical Operator72/4, Logical Operator104/4, Logical Operator103/4, Logical Operator97/4, Logical Operator96/4, Logical Operator116/4, Logical Operator115/4, Logical Operator109/4, Logical Operator108/4, Logical Operator140/4, Logical Operator139/4, Logical Operator133/4, Logical Operator132/4, Logical Operator152/4, Logical Operator151/4, Logical Operator145/4, Logical Operator144/4, Logical Operator164/4, Logical Operator163/4, Logical Operator157/4, Logical Operator156/4, Logical Operator176/4, Logical Operator175/4, Logical Operator169/4, Logical Operator168/4, Logical Operator188/4, Logical Operator183/1
  Address_2(1b)/1 -> Logical Operator182/1, Logical Operator180/3, Logical Operator181/3, Logical Operator185/3, Logical Operator120/3, Logical Operator121/3, Logical Operator125/3, Logical Operator126/3, Logical Operator84/3, Logical Operator85/3, Logical Operator89/3, Logical Operator90/3, Logical Operator/3, Logical Operator1/3, Logical Operator2/3, Logical Operator3/3, Logical Operator18/3, Logical Operator17/3, Logical Operator13/3, Logical Operator9/3, Logical Operator30/3, Logical Operator29/3, Logical Operator25/3, Logical Operator24/3, Logical Operator42/3, Logical Operator41/3, Logical Operator37/3, Logical Operator36/3, Logical Operator54/3, Logical Operator53/3, Logical Operator49/3, Logical Operator48/3, Logical Operator66/3, Logical Operator65/3, Logical Operator61/3, Logical Operator60/3, Logical Operator78/3, Logical Operator77/3, Logical Operator73/3, Logical Operator72/3, Logical Operator102/3, Logical Operator101/3, Logical Operator97/3, Logical Operator96/3, Logical Operator114/3, Logical Operator113/3, Logical Operator109/3, Logical Operator108/3, Logical Operator138/3, Logical Operator137/3, Logical Operator133/3, Logical Operator132/3, Logical Operator150/3, Logical Operator149/3, Logical Operator145/3, Logical Operator144/3, Logical Operator162/3, Logical Operator161/3, Logical Operator157/3, Logical Operator156/3, Logical Operator174/3, Logical Operator173/3, Logical Operator169/3, Logical Operator168/3, Logical Operator186/3
  Bus Selector/1 -> Logical Operator180/1  "<signal1>"
  Bus Selector1/1 -> Logical Operator181/1  "<signal1>"
  Bus Selector2/1 -> Logical Operator185/1  "<signal1>"
  Bus Selector3/1 -> Logical Operator186/1  "<signal1>"
  Bus Selector4/1 -> Logical Operator187/1  "<signal1>"
  Bus Selector5/1 -> Logical Operator188/1  "<signal1>"
  Bus Selector6/1 -> Logical Operator189/1  "<signal1>"
  Bus Selector7/1 -> Logical Operator190/1  "<signal1>"
  Logical Operator190/1 -> Logical Operator191/8
  Logical Operator189/1 -> Logical Operator191/7
  Logical Operator188/1 -> Logical Operator191/6
  Logical Operator187/1 -> Logical Operator191/5
  Logical Operator186/1 -> Logical Operator191/4
  Logical Operator185/1 -> Logical Operator191/3
  Logical Operator181/1 -> Logical Operator191/2
  Logical Operator180/1 -> Logical Operator191/1
  Address_0(1b)/1 -> Logical Operator184/1, Logical Operator180/2, Logical Operator185/2, Logical Operator187/2, Logical Operator120/2, Logical Operator125/2, Logical Operator127/2, Logical Operator129/2, Logical Operator84/2, Logical Operator89/2, Logical Operator91/2, Logical Operator93/2, Logical Operator/2, Logical Operator2/2, Logical Operator4/2, Logical Operator6/2, Logical Operator21/2, Logical Operator19/2, Logical Operator17/2, Logical Operator9/2, Logical Operator33/2, Logical Operator31/2, Logical Operator29/2, Logical Operator24/2, Logical Operator45/2, Logical Operator43/2, Logical Operator41/2, Logical Operator36/2, Logical Operator57/2, Logical Operator55/2, Logical Operator53/2, Logical Operator48/2, Logical Operator69/2, Logical Operator67/2, Logical Operator65/2, Logical Operator60/2, Logical Operator81/2, Logical Operator79/2, Logical Operator77/2, Logical Operator72/2, Logical Operator105/2, Logical Operator103/2, Logical Operator101/2, Logical Operator96/2, Logical Operator117/2, Logical Operator115/2, Logical Operator113/2, Logical Operator108/2, Logical Operator141/2, Logical Operator139/2, Logical Operator137/2, Logical Operator132/2, Logical Operator153/2, Logical Operator151/2, Logical Operator149/2, Logical Operator144/2, Logical Operator165/2, Logical Operator163/2, Logical Operator161/2, Logical Operator156/2, Logical Operator177/2, Logical Operator175/2, Logical Operator173/2, Logical Operator168/2, Logical Operator189/2
